simulink model "CarSim"  (R2019a)
settings: Solver=VariableStepAuto  StartTime=0.0  StopTime=200  RelTol=1e-3
settings Model: Creator=prodani  LastModifiedBy=prodani

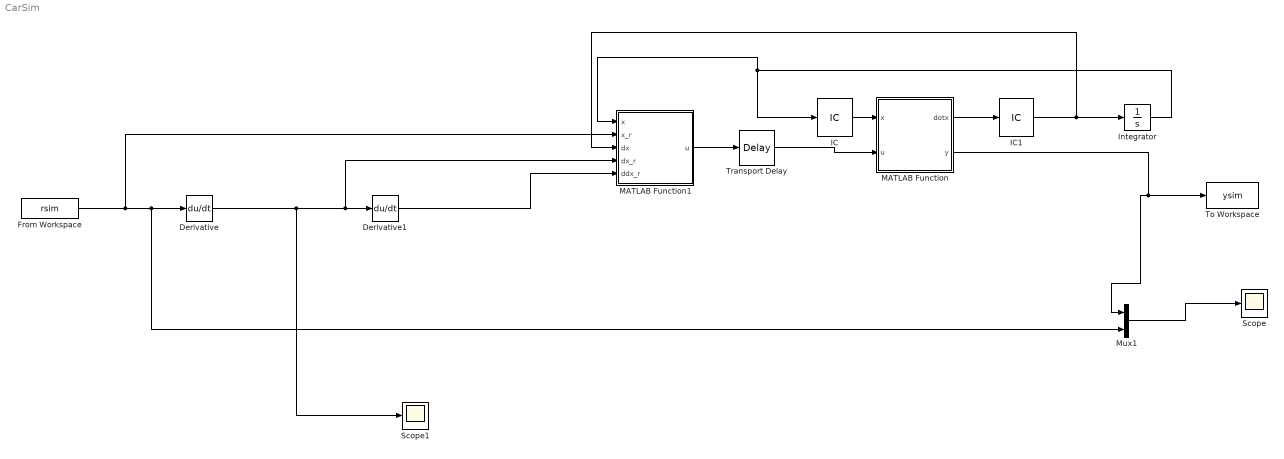
== system CarSim ==
  Derivative : Derivative
  Derivative1 : Derivative
  From Workspace : FromWorkspace  VariableName=rsim  SampleTime=0
  IC : InitialCondition  Value=[0 0 0 1]
  IC1 : InitialCondition  Value=[0 0 0 0]
  Integrator : Integrator  InitialCondition=[0 0 0 1 ]
  MATLAB Function : MATLAB Function  TreatAsAtomicUnit=on
  MATLAB Function1 : MATLAB Function  TreatAsAtomicUnit=on
  Mux1 : Mux  Inputs=2
  Scope : Scope
  Scope1 : Scope
  To Workspace : ToWorkspace  VariableName=ysim  SaveFormat=Structure With Time  SampleTime=-1
  Transport Delay : TransportDelay  DelayTime=0.01
  wires:
  From Workspace/1 -> Derivative/1, Mux1/2, MATLAB Function1/2(x_r)
  Integrator/1 -> MATLAB Function1/1(x), IC/1
  MATLAB Function/1(dotx) -> IC1/1
  Mux1/1 -> Scope/1
  MATLAB Function/2(y) -> Mux1/1, To Workspace/1
  MATLAB Function1/1(u) -> Transport Delay/1
  IC/1 -> MATLAB Function/1(x)
  IC1/1 -> MATLAB Function1/3(dx), Integrator/1
  Derivative/1 -> Scope1/1, Derivative1/1, MATLAB Function1/4(dx_r)
  Derivative1/1 -> MATLAB Function1/5(ddx_r)
  Transport Delay/1 -> MATLAB Function/2(u)

== matlab function CarSim/MATLAB Function1 ==
  data: x input; u output; x_r input; dx input; dx_r input; ddx_r input
function u  = fcn(x,x_r,dx,dx_r,ddx_r)
u=zeros(2,1);
u=inv([-x(4)*sin(x(3)) cos(x(3)); x(4)*cos(x(3)) sin(x(3))])*...
    ((x_r -x(1:2)) + 2*(dx_r - dx(1:2)) + ddx_r);

== matlab function CarSim/MATLAB Function ==
  data: x input; dotx output; u input; y output
function [dotx,y] = fcn(x,u)
dotx=[x(4)*cos(x(3)); x(4)*sin(x(3)); u(1); u(2)];
y = [x(1); x(2) ];
